simulink model "base_model"  (R2020a)
settings: Solver=VariableStepAuto  StartTime=0.0  StopTime=100  RelTol=1e-3
model workspace (MAT data in the model file):
  m = 1000
values from neighbouring files (symbols this model uses):
  ci = 577.1044    [rocky_constants.m]
  g = 9.8    [rocky_constants.m]
  ji = 788.7322    [rocky_constants.m]
  jp = -30.4904    [rocky_constants.m]
  ki = -8132    [rocky_constants.m]
  kmotor = .0025    (= 0.0025)    [rocky_constants.m]
  kp = -1739    [rocky_constants.m]
  l = 0.4822    [rocky_constants.m]
  tau = .103    (= 0.103)    [rocky_constants.m]
settings Model: Creator=clee1  LastModifiedBy=mkazazic

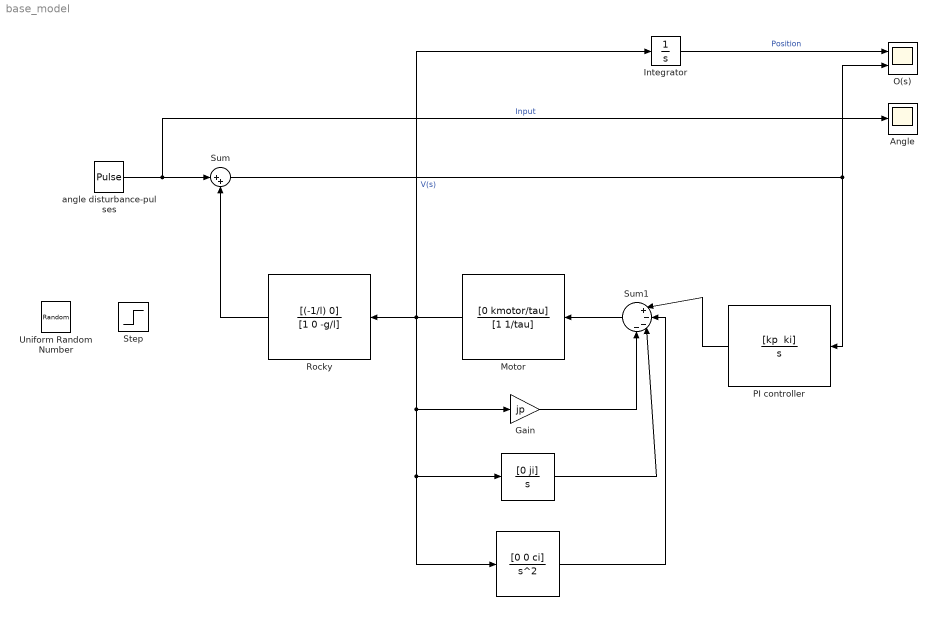
== system base_model ==
  " " : TransferFcn  Numerator=[0 ji]  Denominator=[1 0]
  "  " : TransferFcn  Numerator=[0 0 ci]  Denominator=[1 0 0]
  Angle : Scope
  Gain : Gain  Gain=jp
  Integrator : Integrator
  Motor : TransferFcn  Numerator=[0 kmotor/tau]  Denominator=[1 1/tau]
  O(s) : Scope  NumInputPorts=2
  PI controller : TransferFcn  Numerator="[kp  ki]"  Denominator=[1 0 ]
  Rocky : TransferFcn  Numerator=[(-1/l) 0]  Denominator=[1 0 -g/l]
  Step : Step  After=.1  SampleTime=0
  Sum : Sum  Inputs=|++
  Sum1 : Sum  Inputs=|+---
  Uniform Random Number : UniformRandomNumber  SampleTime=20
  angle disturbance-pulses : DiscretePulseGenerator  PulseType=Time based  Amplitude=.1  Period=10
  wires:
  Motor/1 -> "  "/1, " "/1, Gain/1, Integrator/1, Rocky/1  "V(s)"
  Sum/1 -> PI controller/1, O(s)/2
  angle disturbance-pulses/1 -> Angle/1, Sum/1  "Input"
  Gain/1 -> Sum1/4
  " "/1 -> Sum1/3
  "  "/1 -> Sum1/2
  Sum1/1 -> Motor/1
  Rocky/1 -> Sum/2
  PI controller/1 -> Sum1/1
  Integrator/1 -> O(s)/1  "Position"
